simulink model "BaseControl"  (R2021a)
settings: Solver=FixedStepAuto  StartTime=0.0  StopTime=20  FixedStep=10/1000  RelTol=1e-3  EnableMultiTasking=on
values from neighbouring files (symbols this model uses):
  delay = 0    [LoadModel.m]
  den = conv([1 1],[0.5^2 1.4*0.5 1])    [LoadModel.m]
  num = 1    [LoadModel.m]
settings Model: Creator=g.reynosomeza  LastModifiedBy=mluser
settings SolverCC: AlgebraicLoopSolver=TrustRegion
settings DataIOCC: LimitDataPoints=on  SaveFormat=Array  ReturnWorkspaceOutputs=off
settings OptimizationCC: LifeSpan=inf
settings DebuggingCC: AlgebraicLoopMsg=none  ArtificialAlgebraicLoopMsg=none  SolverPrmCheckMsg=warning  SFUnexpectedBacktrackingDiag=warning  SFNoUnconditionalDefaultTransitionDiag=warning  SFExecutionAtInitializationDiag=none  SFMachineParentedDataDiag=warning  ArithmeticOperatorsInVariantConditions=warning
settings HardwareCC: ProdBitPerPointer=32  ProdBitPerSizeT=32  ProdBitPerPtrDiffT=32  ProdLargestAtomicFloat=None  ProdIntDivRoundTo=Undefined  ProdEndianess=Unspecified  ProdWordSize=32  ProdHWDeviceType=32-bit Generic
settings ModelReferenceCC: PropagateSignalLabelsOutOfModel=off
settings SFSimCC: SimUseLocalCustomCode=off  CustomCodeUndefinedFunction=UseInterfaceOnly
settings RTWCC: RTWUseLocalCustomCode=off
settings CodeAppCC: StateflowObjectComments=on
settings GRTTargetCC: TargetLangStandard=C89/C90 (ANSI)
settings ConfigComp: CovMetricSettings=dw  CovSaveCumulativeToWorkspaceVar=on  CovSaveSingleToWorkspaceVar=on  CovExternalEMLEnable=off  CovSFcnEnable=off

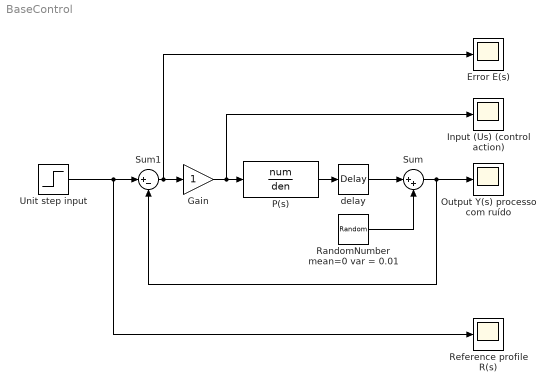
== system BaseControl ==
  Error E(s) : Scope
  Gain : Gain
  Input (Us) (control action) : Scope
  Output Y(s) processo com ruído : Scope
  P(s) : TransferFcn  Numerator=num  Denominator=den
  RandomNumber mean=0 var = 0.01 : RandomNumber  Variance=0.001  SampleTime=10/1000
  Reference profile R(s) : Scope
  Sum : Sum  Inputs=|++
  Sum1 : Sum  Inputs=|+-
  Unit step input : Step  Time=5  SampleTime=0
  delay : TransportDelay  DelayTime=delay
  wires:
  Unit step input/1 -> Sum1/1, Reference profile R(s)/1
  P(s)/1 -> delay/1
  delay/1 -> Sum/1
  RandomNumber mean=0 var = 0.01/1 -> Sum/2
  Sum/1 -> Sum1/2, Output Y(s) processo com ruído/1
  Sum1/1 -> Gain/1, Error E(s)/1
  Gain/1 -> P(s)/1, Input (Us) (control action)/1
